simulink model "flame"  (R2024b)
settings: Solver=VariableStepAuto  StartTime=0.0  StopTime=10.0  RelTol=1e-3
libraries: taXlibrary x6
settings Model: Creator=Tanguy  LastModifiedBy=Tanguy

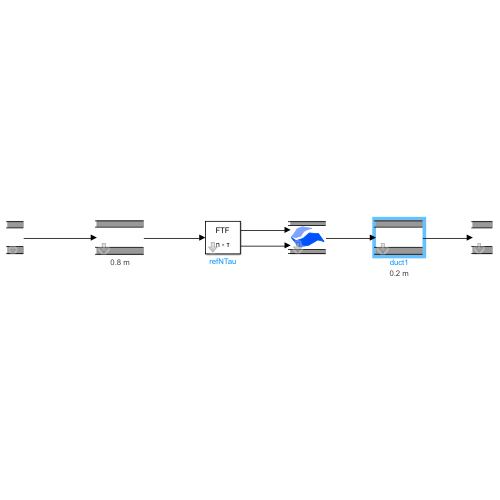
[thumbnail: Simulink's stored preview of the top-level diagram]
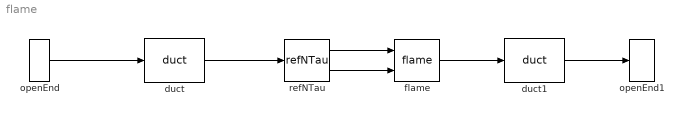
== system flame ==
  duct : taXlibrary/duct  element=Duct  l=0.8  phi_active=on  T_active=on  omega_active=on  omegafree_active=on  posup=[]  posdn=[]  sensorPositions=[]  order=3  minres=40
      settings: AttributesFormatString=%<l> m
  duct1 : taXlibrary/duct  element=Duct  l=0.2  phi_active=on  T_active=on  omega_active=on  omegafree_active=on  posup=[]  posdn=[]  sensorPositions=[]  order=3  minres=40
      settings: AttributesFormatString=%<l> m
  flame : taXlibrary/flame  element=symAreaChangeRankineHugoniot  nRef=1  Version=constant cp, classic Rankine-Hugoniot, f and g only  Aratio=1.2  Tratio=5  kratio=.921  fuel=H2  Hu=55.5e6  a_CaHb=1  b_CaHb=4  pos=[]
  openEnd : taXlibrary/openEnd  element=openEnd  loc=Upstream  Area=1  Mach=0.05  rho=1.2  c_sound=340  kappa=1.4  Mmol=29  alpha=0.1  pos=[]
  openEnd1 : taXlibrary/openEnd  element=openEnd  loc=Downstream  Area=[]  Mach=[]  rho=[]  c_sound=[]  kappa=[]  Mmol=[]  alpha=[]  pos=[]
  refNTau : taXlibrary/refNTau  element=referenceGeneral  n=0.1  tau=0.0005  active=on  filename=FTF_ntau.m  modelname=0  pos=[]
  wires:
  openEnd/1 -> duct/1
  duct/1 -> refNTau/1
  refNTau/1 -> flame/1
  refNTau/2 -> flame/2
  duct1/1 -> openEnd1/1
  flame/1 -> duct1/1
